simulink model "IOControls"  (R2019b)
settings: configuration reference "ConfigSet_IOControls_Reference" (kept outside this file)
model workspace (MAT data in the model file):
  SampleTime = 0.05
libraries: IOStateMachinesLib x274, SignalGeneratorsLib x1, simulink x1
(part 3 of 10)

== system IOControls/ForEachVehicle/IOControls/Non-CabControl/EDBPanel ==
  ModelInputs : Inport
  Initialise : Inport  Port=2
  BC_Inputs : BusCreator  Inputs=3
  BC_MCBTrip : BusCreator  Inputs=1
  BS_Control1 : BusSelector  OutputSignals=PantographIsolationCock
  BS_Control2 : BusSelector  OutputSignals=VCBIsolationCock
  BS_Control3 : BusSelector  OutputSignals=ORDPlunger
  MCBTripGround : Ground
  ORDPlunger : Subsystem  mask{InitState=0, ControlStates=[0,1], OnStateValue=1, OffStateValue=0}
      mask prompts: InitState "Initial State"; ControlStates "Software State Values"; OnStateValue "On State Value"; OffStateValue "Off State Value"
  PantographIsolationCock : Subsystem  mask{InitState=1, ControlStates=[0,1], OnStateValue=1, OffStateValue=0}
      mask prompts: InitState "Initial State"; ControlStates "Software State Values"; OnStateValue "On State Value"; OffStateValue "Off State Value"
  VCBIsolationCock : Subsystem  mask{InitState=1, ControlStates=[0,1], OnStateValue=1, OffStateValue=0}
      mask prompts: InitState "Initial State"; ControlStates "Software State Values"; OnStateValue "On State Value"; OffStateValue "Off State Value"
  TierControlsInputs : Outport  VectorParamsAs1DForOutWhenUnconnected=off
  TierControlsMCBTrip : Outport  Port=2  VectorParamsAs1DForOutWhenUnconnected=off
  wires:
  MCBTripGround/1 -> BC_MCBTrip/1
  BC_MCBTrip/1 -> TierControlsMCBTrip/1  "EDBPanel"
  BC_Inputs/1 -> TierControlsInputs/1  "EDBPanel"
  ModelInputs/1 -> BS_Control1/1, BS_Control2/1, BS_Control3/1
  BS_Control1/1 -> PantographIsolationCock/1(InputControl)  "<PantographIsolationCock>"
  Initialise/1 -> PantographIsolationCock/2(Initialise), VCBIsolationCock/2(Initialise), ORDPlunger/2(Initialise)
  PantographIsolationCock/1(InputState) -> BC_Inputs/1  "PantographIsolationCock"
  BS_Control2/1 -> VCBIsolationCock/1(InputControl)  "<VCBIsolationCock>"
  VCBIsolationCock/1(InputState) -> BC_Inputs/2  "VCBIsolationCock"
  BS_Control3/1 -> ORDPlunger/1(InputControl)  "<ORDPlunger>"
  ORDPlunger/1(InputState) -> BC_Inputs/3  "ORDPlunger"

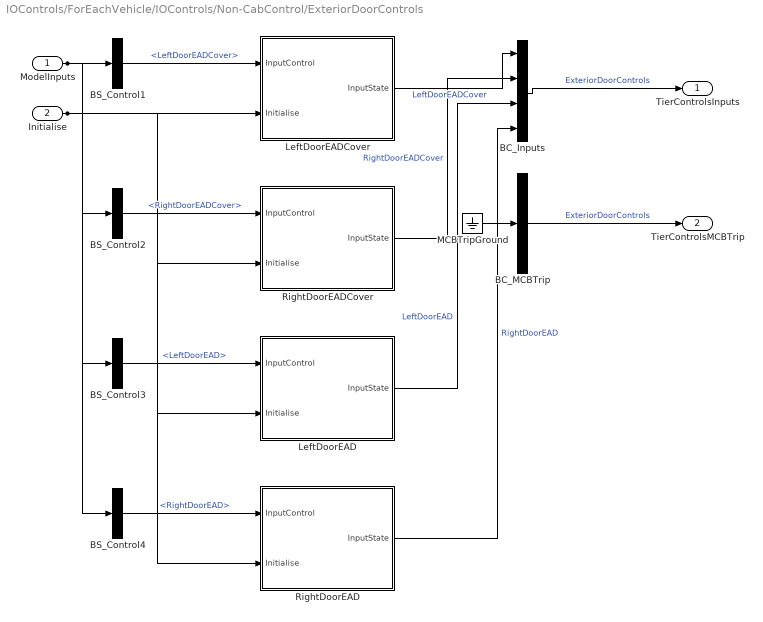
== system IOControls/ForEachVehicle/IOControls/Non-CabControl/ExteriorDoorControls ==
  ModelInputs : Inport
  Initialise : Inport  Port=2
  BC_Inputs : BusCreator  Inputs=4
  BC_MCBTrip : BusCreator  Inputs=1
  BS_Control1 : BusSelector  OutputSignals=LeftDoorEADCover
  BS_Control2 : BusSelector  OutputSignals=RightDoorEADCover
  BS_Control3 : BusSelector  OutputSignals=LeftDoorEAD
  BS_Control4 : BusSelector  OutputSignals=RightDoorEAD
  LeftDoorEAD : Subsystem  mask{InitState=0, ControlStates=[0,1], OnStateValue=1, OffStateValue=0}
      mask prompts: InitState "Initial State"; ControlStates "Software State Values"; OnStateValue "On State Value"; OffStateValue "Off State Value"
  LeftDoorEADCover : Subsystem  mask{InitState=0, ControlStates=[0,1], OnStateValue=1, OffStateValue=0}
      mask prompts: InitState "Initial State"; ControlStates "Software State Values"; OnStateValue "On State Value"; OffStateValue "Off State Value"
  MCBTripGround : Ground
  RightDoorEAD : Subsystem  mask{InitState=0, ControlStates=[0,1], OnStateValue=1, OffStateValue=0}
      mask prompts: InitState "Initial State"; ControlStates "Software State Values"; OnStateValue "On State Value"; OffStateValue "Off State Value"
  RightDoorEADCover : Subsystem  mask{InitState=0, ControlStates=[0,1], OnStateValue=1, OffStateValue=0}
      mask prompts: InitState "Initial State"; ControlStates "Software State Values"; OnStateValue "On State Value"; OffStateValue "Off State Value"
  TierControlsInputs : Outport  VectorParamsAs1DForOutWhenUnconnected=off
  TierControlsMCBTrip : Outport  Port=2  VectorParamsAs1DForOutWhenUnconnected=off
  wires:
  MCBTripGround/1 -> BC_MCBTrip/1
  BC_MCBTrip/1 -> TierControlsMCBTrip/1  "ExteriorDoorControls"
  BC_Inputs/1 -> TierControlsInputs/1  "ExteriorDoorControls"
  ModelInputs/1 -> BS_Control1/1, BS_Control2/1, BS_Control3/1, BS_Control4/1
  BS_Control1/1 -> LeftDoorEADCover/1(InputControl)  "<LeftDoorEADCover>"
  Initialise/1 -> LeftDoorEADCover/2(Initialise), RightDoorEADCover/2(Initialise), LeftDoorEAD/2(Initialise), RightDoorEAD/2(Initialise)
  LeftDoorEADCover/1(InputState) -> BC_Inputs/1  "LeftDoorEADCover"
  BS_Control2/1 -> RightDoorEADCover/1(InputControl)  "<RightDoorEADCover>"
  RightDoorEADCover/1(InputState) -> BC_Inputs/2  "RightDoorEADCover"
  BS_Control3/1 -> LeftDoorEAD/1(InputControl)  "<LeftDoorEAD>"
  LeftDoorEAD/1(InputState) -> BC_Inputs/3  "LeftDoorEAD"
  BS_Control4/1 -> RightDoorEAD/1(InputControl)  "<RightDoorEAD>"
  RightDoorEAD/1(InputState) -> BC_Inputs/4  "RightDoorEAD"

== system IOControls/ForEachVehicle/IOControls/Non-CabControl/ExteriorLights ==
  ModelInputs : Inport
  Initialise : Inport  Port=2
  BC_Inputs : BusCreator  Inputs=1
  BC_MCBTrip : BusCreator  Inputs=1
  InitialiseTerminator : Terminator
  InputsGround : Ground
  MCBTripGround : Ground
  ModelInputsTerminator : Terminator
  TierControlsInputs : Outport  VectorParamsAs1DForOutWhenUnconnected=off
  TierControlsMCBTrip : Outport  Port=2  VectorParamsAs1DForOutWhenUnconnected=off
  wires:
  MCBTripGround/1 -> BC_MCBTrip/1
  InputsGround/1 -> BC_Inputs/1
  Initialise/1 -> InitialiseTerminator/1
  ModelInputs/1 -> ModelInputsTerminator/1
  BC_MCBTrip/1 -> TierControlsMCBTrip/1  "ExteriorLights"
  BC_Inputs/1 -> TierControlsInputs/1  "ExteriorLights"

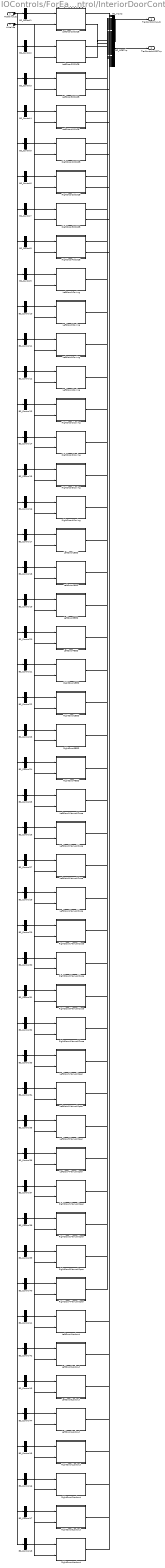
== system IOControls/ForEachVehicle/IOControls/Non-CabControl/InteriorDoorControls ==
  ModelInputs : Inport
  Initialise : Inport  Port=2
  BC_Inputs : BusCreator  Inputs=48
  BC_MCBTrip : BusCreator  Inputs=8
  BS_Control1 : BusSelector  OutputSignals=LeftDoor1DCUCB
  BS_Control10 : BusSelector  OutputSignals=LeftDoor2Coving
  BS_Control11 : BusSelector  OutputSignals=LeftDoor3Coving
  BS_Control12 : BusSelector  OutputSignals=LeftDoor4Coving
  BS_Control13 : BusSelector  OutputSignals=RightDoor1Coving
  BS_Control14 : BusSelector  OutputSignals=RightDoor2Coving
  BS_Control15 : BusSelector  OutputSignals=RightDoor3Coving
  BS_Control16 : BusSelector  OutputSignals=RightDoor4Coving
  BS_Control17 : BusSelector  OutputSignals=LeftDoor1EED
  BS_Control18 : BusSelector  OutputSignals=LeftDoor2EED
  BS_Control19 : BusSelector  OutputSignals=LeftDoor3EED
  BS_Control2 : BusSelector  OutputSignals=LeftDoor2DCUCB
  BS_Control20 : BusSelector  OutputSignals=LeftDoor4EED
  BS_Control21 : BusSelector  OutputSignals=RightDoor1EED
  BS_Control22 : BusSelector  OutputSignals=RightDoor2EED
  BS_Control23 : BusSelector  OutputSignals=RightDoor3EED
  BS_Control24 : BusSelector  OutputSignals=RightDoor4EED
  BS_Control25 : BusSelector  OutputSignals=LeftDoor1ManualClose
  BS_Control26 : BusSelector  OutputSignals=LeftDoor2ManualClose
  BS_Control27 : BusSelector  OutputSignals=LeftDoor3ManualClose
  BS_Control28 : BusSelector  OutputSignals=LeftDoor4ManualClose
  BS_Control29 : BusSelector  OutputSignals=RightDoor1ManualClose
  BS_Control3 : BusSelector  OutputSignals=LeftDoor3DCUCB
  BS_Control30 : BusSelector  OutputSignals=RightDoor2ManualClose
  BS_Control31 : BusSelector  OutputSignals=RightDoor3ManualClose
  BS_Control32 : BusSelector  OutputSignals=RightDoor4ManualClose
  BS_Control33 : BusSelector  OutputSignals=LeftDoor1ManualOpen
  BS_Control34 : BusSelector  OutputSignals=LeftDoor2ManualOpen
  BS_Control35 : BusSelector  OutputSignals=LeftDoor3ManualOpen
  BS_Control36 : BusSelector  OutputSignals=LeftDoor4ManualOpen
  BS_Control37 : BusSelector  OutputSignals=RightDoor1ManualOpen
  BS_Control38 : BusSelector  OutputSignals=RightDoor2ManualOpen
  BS_Control39 : BusSelector  OutputSignals=RightDoor3ManualOpen
  BS_Control4 : BusSelector  OutputSignals=LeftDoor4DCUCB
  BS_Control40 : BusSelector  OutputSignals=RightDoor4ManualOpen
  BS_Control41 : BusSelector  OutputSignals=LeftDoor1Lockout
  BS_Control42 : BusSelector  OutputSignals=LeftDoor2Lockout
  BS_Control43 : BusSelector  OutputSignals=LeftDoor3Lockout
  BS_Control44 : BusSelector  OutputSignals=LeftDoor4Lockout
  BS_Control45 : BusSelector  OutputSignals=RightDoor1Lockout
  BS_Control46 : BusSelector  OutputSignals=RightDoor2Lockout
  BS_Control47 : BusSelector  OutputSignals=RightDoor3Lockout
  BS_Control48 : BusSelector  OutputSignals=RightDoor4Lockout
  BS_Control5 : BusSelector  OutputSignals=RightDoor1DCUCB
  BS_Control6 : BusSelector  OutputSignals=RightDoor2DCUCB
  BS_Control7 : BusSelector  OutputSignals=RightDoor3DCUCB
  BS_Control8 : BusSelector  OutputSignals=RightDoor4DCUCB
  BS_Control9 : BusSelector  OutputSignals=LeftDoor1Coving
  LeftDoor1Coving : Subsystem  mask{InitState=0, ControlStates=[0,1], OnStateValue=1, OffStateValue=0}
      mask prompts: InitState "Initial State"; ControlStates "Software State Values"; OnStateValue "On State Value"; OffStateValue "Off State Value"
  LeftDoor1DCUCB : Subsystem  mask{InitState=1, ControlStates=[0,1], OnStateValue=1, OffStateValue=0}
      mask prompts: InitState "Initial State"; ControlStates "Software State Values"; OnStateValue "On State Value"; OffStateValue "Off State Value"
  LeftDoor1EED : Subsystem  mask{InitState=0, ControlStates=[0,1], OnStateValue=1, OffStateValue=0}
      mask prompts: InitState "Initial State"; ControlStates "Software State Values"; OnStateValue "On State Value"; OffStateValue "Off State Value"
  LeftDoor1Lockout : Subsystem  mask{InitState=0, ControlStates=[0,1], OnStateValue=1, OffStateValue=0}
      mask prompts: InitState "Initial State"; ControlStates "Software State Values"; OnStateValue "On State Value"; OffStateValue "Off State Value"
  LeftDoor1ManualClose : Subsystem  mask{InitState=0, ControlStates=[0,1], OnStateValue=1, OffStateValue=0}
      mask prompts: InitState "Initial State"; ControlStates "Software State Values"; OnStateValue "On State Value"; OffStateValue "Off State Value"
  LeftDoor1ManualOpen : Subsystem  mask{InitState=0, ControlStates=[0,1], OnStateValue=1, OffStateValue=0}
      mask prompts: InitState "Initial State"; ControlStates "Software State Values"; OnStateValue "On State Value"; OffStateValue "Off State Value"
  LeftDoor2Coving : Subsystem  mask{InitState=0, ControlStates=[0,1], OnStateValue=1, OffStateValue=0}
      mask prompts: InitState "Initial State"; ControlStates "Software State Values"; OnStateValue "On State Value"; OffStateValue "Off State Value"
  LeftDoor2DCUCB : Subsystem  mask{InitState=1, ControlStates=[0,1], OnStateValue=1, OffStateValue=0}
      mask prompts: InitState "Initial State"; ControlStates "Software State Values"; OnStateValue "On State Value"; OffStateValue "Off State Value"
  LeftDoor2EED : Subsystem  mask{InitState=0, ControlStates=[0,1], OnStateValue=1, OffStateValue=0}
      mask prompts: InitState "Initial State"; ControlStates "Software State Values"; OnStateValue "On State Value"; OffStateValue "Off State Value"
  LeftDoor2Lockout : Subsystem  mask{InitState=0, ControlStates=[0,1], OnStateValue=1, OffStateValue=0}
      mask prompts: InitState "Initial State"; ControlStates "Software State Values"; OnStateValue "On State Value"; OffStateValue "Off State Value"
  LeftDoor2ManualClose : Subsystem  mask{InitState=0, ControlStates=[0,1], OnStateValue=1, OffStateValue=0}
      mask prompts: InitState "Initial State"; ControlStates "Software State Values"; OnStateValue "On State Value"; OffStateValue "Off State Value"
  LeftDoor2ManualOpen : Subsystem  mask{InitState=0, ControlStates=[0,1], OnStateValue=1, OffStateValue=0}
      mask prompts: InitState "Initial State"; ControlStates "Software State Values"; OnStateValue "On State Value"; OffStateValue "Off State Value"
  LeftDoor3Coving : Subsystem  mask{InitState=0, ControlStates=[0,1], OnStateValue=1, OffStateValue=0}
      mask prompts: InitState "Initial State"; ControlStates "Software State Values"; OnStateValue "On State Value"; OffStateValue "Off State Value"
  LeftDoor3DCUCB : Subsystem  mask{InitState=1, ControlStates=[0,1], OnStateValue=1, OffStateValue=0}
      mask prompts: InitState "Initial State"; ControlStates "Software State Values"; OnStateValue "On State Value"; OffStateValue "Off State Value"
  LeftDoor3EED : Subsystem  mask{InitState=0, ControlStates=[0,1], OnStateValue=1, OffStateValue=0}
      mask prompts: InitState "Initial State"; ControlStates "Software State Values"; OnStateValue "On State Value"; OffStateValue "Off State Value"
  LeftDoor3Lockout : Subsystem  mask{InitState=0, ControlStates=[0,1], OnStateValue=1, OffStateValue=0}
      mask prompts: InitState "Initial State"; ControlStates "Software State Values"; OnStateValue "On State Value"; OffStateValue "Off State Value"
  LeftDoor3ManualClose : Subsystem  mask{InitState=0, ControlStates=[0,1], OnStateValue=1, OffStateValue=0}
      mask prompts: InitState "Initial State"; ControlStates "Software State Values"; OnStateValue "On State Value"; OffStateValue "Off State Value"
  LeftDoor3ManualOpen : Subsystem  mask{InitState=0, ControlStates=[0,1], OnStateValue=1, OffStateValue=0}
      mask prompts: InitState "Initial State"; ControlStates "Software State Values"; OnStateValue "On State Value"; OffStateValue "Off State Value"
  LeftDoor4Coving : Subsystem  mask{InitState=0, ControlStates=[0,1], OnStateValue=1, OffStateValue=0}
      mask prompts: InitState "Initial State"; ControlStates "Software State Values"; OnStateValue "On State Value"; OffStateValue "Off State Value"
  LeftDoor4DCUCB : Subsystem  mask{InitState=1, ControlStates=[0,1], OnStateValue=1, OffStateValue=0}
      mask prompts: InitState "Initial State"; ControlStates "Software State Values"; OnStateValue "On State Value"; OffStateValue "Off State Value"
  LeftDoor4EED : Subsystem  mask{InitState=0, ControlStates=[0,1], OnStateValue=1, OffStateValue=0}
      mask prompts: InitState "Initial State"; ControlStates "Software State Values"; OnStateValue "On State Value"; OffStateValue "Off State Value"
  LeftDoor4Lockout : Subsystem  mask{InitState=0, ControlStates=[0,1], OnStateValue=1, OffStateValue=0}
      mask prompts: InitState "Initial State"; ControlStates "Software State Values"; OnStateValue "On State Value"; OffStateValue "Off State Value"
  LeftDoor4ManualClose : Subsystem  mask{InitState=0, ControlStates=[0,1], OnStateValue=1, OffStateValue=0}
      mask prompts: InitState "Initial State"; ControlStates "Software State Values"; OnStateValue "On State Value"; OffStateValue "Off State Value"
  LeftDoor4ManualOpen : Subsystem  mask{InitState=0, ControlStates=[0,1], OnStateValue=1, OffStateValue=0}
      mask prompts: InitState "Initial State"; ControlStates "Software State Values"; OnStateValue "On State Value"; OffStateValue "Off State Value"
  RightDoor1Coving : Subsystem  mask{InitState=0, ControlStates=[0,1], OnStateValue=1, OffStateValue=0}
      mask prompts: InitState "Initial State"; ControlStates "Software State Values"; OnStateValue "On State Value"; OffStateValue "Off State Value"
  RightDoor1DCUCB : Subsystem  mask{InitState=1, ControlStates=[0,1], OnStateValue=1, OffStateValue=0}
      mask prompts: InitState "Initial State"; ControlStates "Software State Values"; OnStateValue "On State Value"; OffStateValue "Off State Value"
  RightDoor1EED : Subsystem  mask{InitState=0, ControlStates=[0,1], OnStateValue=1, OffStateValue=0}
      mask prompts: InitState "Initial State"; ControlStates "Software State Values"; OnStateValue "On State Value"; OffStateValue "Off State Value"
  RightDoor1Lockout : Subsystem  mask{InitState=0, ControlStates=[0,1], OnStateValue=1, OffStateValue=0}
      mask prompts: InitState "Initial State"; ControlStates "Software State Values"; OnStateValue "On State Value"; OffStateValue "Off State Value"
  RightDoor1ManualClose : Subsystem  mask{InitState=0, ControlStates=[0,1], OnStateValue=1, OffStateValue=0}
      mask prompts: InitState "Initial State"; ControlStates "Software State Values"; OnStateValue "On State Value"; OffStateValue "Off State Value"
  RightDoor1ManualOpen : Subsystem  mask{InitState=0, ControlStates=[0,1], OnStateValue=1, OffStateValue=0}
      mask prompts: InitState "Initial State"; ControlStates "Software State Values"; OnStateValue "On State Value"; OffStateValue "Off State Value"
  RightDoor2Coving : Subsystem  mask{InitState=0, ControlStates=[0,1], OnStateValue=1, OffStateValue=0}
      mask prompts: InitState "Initial State"; ControlStates "Software State Values"; OnStateValue "On State Value"; OffStateValue "Off State Value"
  RightDoor2DCUCB : Subsystem  mask{InitState=1, ControlStates=[0,1], OnStateValue=1, OffStateValue=0}
      mask prompts: InitState "Initial State"; ControlStates "Software State Values"; OnStateValue "On State Value"; OffStateValue "Off State Value"
  RightDoor2EED : Subsystem  mask{InitState=0, ControlStates=[0,1], OnStateValue=1, OffStateValue=0}
      mask prompts: InitState "Initial State"; ControlStates "Software State Values"; OnStateValue "On State Value"; OffStateValue "Off State Value"
  RightDoor2Lockout : Subsystem  mask{InitState=0, ControlStates=[0,1], OnStateValue=1, OffStateValue=0}
      mask prompts: InitState "Initial State"; ControlStates "Software State Values"; OnStateValue "On State Value"; OffStateValue "Off State Value"
  RightDoor2ManualClose : Subsystem  mask{InitState=0, ControlStates=[0,1], OnStateValue=1, OffStateValue=0}
      mask prompts: InitState "Initial State"; ControlStates "Software State Values"; OnStateValue "On State Value"; OffStateValue "Off State Value"
  RightDoor2ManualOpen : Subsystem  mask{InitState=0, ControlStates=[0,1], OnStateValue=1, OffStateValue=0}
      mask prompts: InitState "Initial State"; ControlStates "Software State Values"; OnStateValue "On State Value"; OffStateValue "Off State Value"
  RightDoor3Coving : Subsystem  mask{InitState=0, ControlStates=[0,1], OnStateValue=1, OffStateValue=0}
      mask prompts: InitState "Initial State"; ControlStates "Software State Values"; OnStateValue "On State Value"; OffStateValue "Off State Value"
  RightDoor3DCUCB : Subsystem  mask{InitState=1, ControlStates=[0,1], OnStateValue=1, OffStateValue=0}
      mask prompts: InitState "Initial State"; ControlStates "Software State Values"; OnStateValue "On State Value"; OffStateValue "Off State Value"
  RightDoor3EED : Subsystem  mask{InitState=0, ControlStates=[0,1], OnStateValue=1, OffStateValue=0}
      mask prompts: InitState "Initial State"; ControlStates "Software State Values"; OnStateValue "On State Value"; OffStateValue "Off State Value"
  RightDoor3Lockout : Subsystem  mask{InitState=0, ControlStates=[0,1], OnStateValue=1, OffStateValue=0}
      mask prompts: InitState "Initial State"; ControlStates "Software State Values"; OnStateValue "On State Value"; OffStateValue "Off State Value"
  RightDoor3ManualClose : Subsystem  mask{InitState=0, ControlStates=[0,1], OnStateValue=1, OffStateValue=0}
      mask prompts: InitState "Initial State"; ControlStates "Software State Values"; OnStateValue "On State Value"; OffStateValue "Off State Value"
  RightDoor3ManualOpen : Subsystem  mask{InitState=0, ControlStates=[0,1], OnStateValue=1, OffStateValue=0}
      mask prompts: InitState "Initial State"; ControlStates "Software State Values"; OnStateValue "On State Value"; OffStateValue "Off State Value"
  RightDoor4Coving : Subsystem  mask{InitState=0, ControlStates=[0,1], OnStateValue=1, OffStateValue=0}
      mask prompts: InitState "Initial State"; ControlStates "Software State Values"; OnStateValue "On State Value"; OffStateValue "Off State Value"
  RightDoor4DCUCB : Subsystem  mask{InitState=1, ControlStates=[0,1], OnStateValue=1, OffStateValue=0}
      mask prompts: InitState "Initial State"; ControlStates "Software State Values"; OnStateValue "On State Value"; OffStateValue "Off State Value"
  RightDoor4EED : Subsystem  mask{InitState=0, ControlStates=[0,1], OnStateValue=1, OffStateValue=0}
      mask prompts: InitState "Initial State"; ControlStates "Software State Values"; OnStateValue "On State Value"; OffStateValue "Off State Value"
  RightDoor4Lockout : Subsystem  mask{InitState=0, ControlStates=[0,1], OnStateValue=1, OffStateValue=0}
      mask prompts: InitState "Initial State"; ControlStates "Software State Values"; OnStateValue "On State Value"; OffStateValue "Off State Value"
  RightDoor4ManualClose : Subsystem  mask{InitState=0, ControlStates=[0,1], OnStateValue=1, OffStateValue=0}
      mask prompts: InitState "Initial State"; ControlStates "Software State Values"; OnStateValue "On State Value"; OffStateValue "Off State Value"
  RightDoor4ManualOpen : Subsystem  mask{InitState=0, ControlStates=[0,1], OnStateValue=1, OffStateValue=0}
      mask prompts: InitState "Initial State"; ControlStates "Software State Values"; OnStateValue "On State Value"; OffStateValue "Off State Value"
  TierControlsInputs : Outport  VectorParamsAs1DForOutWhenUnconnected=off
  TierControlsMCBTrip : Outport  Port=2  VectorParamsAs1DForOutWhenUnconnected=off
  wires:
  BC_MCBTrip/1 -> TierControlsMCBTrip/1  "InteriorDoorControls"
  BC_Inputs/1 -> TierControlsInputs/1  "InteriorDoorControls"
  ModelInputs/1 -> BS_Control1/1, BS_Control2/1, BS_Control3/1, BS_Control4/1, BS_Control5/1, BS_Control6/1, BS_Control7/1, BS_Control8/1, BS_Control9/1, BS_Control10/1, BS_Control11/1, BS_Control12/1, BS_Control13/1, BS_Control14/1, BS_Control15/1, BS_Control16/1, BS_Control17/1, BS_Control18/1, BS_Control19/1, BS_Control20/1, BS_Control21/1, BS_Control22/1, BS_Control23/1, BS_Control24/1, BS_Control25/1, BS_Control26/1, BS_Control27/1, BS_Control28/1, BS_Control29/1, BS_Control30/1, BS_Control31/1, BS_Control32/1, BS_Control33/1, BS_Control34/1, BS_Control35/1, BS_Control36/1, BS_Control37/1, BS_Control38/1, BS_Control39/1, BS_Control40/1, BS_Control41/1, BS_Control42/1, BS_Control43/1, BS_Control44/1, BS_Control45/1, BS_Control46/1, BS_Control47/1, BS_Control48/1
  BS_Control1/1 -> LeftDoor1DCUCB/1(MCBControl)  "<LeftDoor1DCUCB>"
  Initialise/1 -> LeftDoor1DCUCB/2(Initialise), LeftDoor2DCUCB/2(Initialise), LeftDoor3DCUCB/2(Initialise), LeftDoor4DCUCB/2(Initialise), RightDoor1DCUCB/2(Initialise), RightDoor2DCUCB/2(Initialise), RightDoor3DCUCB/2(Initialise), RightDoor4DCUCB/2(Initialise), LeftDoor1Coving/2(Initialise), LeftDoor2Coving/2(Initialise), LeftDoor3Coving/2(Initialise), LeftDoor4Coving/2(Initialise), RightDoor1Coving/2(Initialise), RightDoor2Coving/2(Initialise), RightDoor3Coving/2(Initialise), RightDoor4Coving/2(Initialise), LeftDoor1EED/2(Initialise), LeftDoor2EED/2(Initialise), LeftDoor3EED/2(Initialise), LeftDoor4EED/2(Initialise), RightDoor1EED/2(Initialise), RightDoor2EED/2(Initialise), RightDoor3EED/2(Initialise), RightDoor4EED/2(Initialise), LeftDoor1ManualClose/2(Initialise), LeftDoor2ManualClose/2(Initialise), LeftDoor3ManualClose/2(Initialise), LeftDoor4ManualClose/2(Initialise), RightDoor1ManualClose/2(Initialise), RightDoor2ManualClose/2(Initialise), RightDoor3ManualClose/2(Initialise), RightDoor4ManualClose/2(Initialise), LeftDoor1ManualOpen/2(Initialise), LeftDoor2ManualOpen/2(Initialise), LeftDoor3ManualOpen/2(Initialise), LeftDoor4ManualOpen/2(Initialise), RightDoor1ManualOpen/2(Initialise), RightDoor2ManualOpen/2(Initialise), RightDoor3ManualOpen/2(Initialise), RightDoor4ManualOpen/2(Initialise), LeftDoor1Lockout/2(Initialise), LeftDoor2Lockout/2(Initialise), LeftDoor3Lockout/2(Initialise), LeftDoor4Lockout/2(Initialise), RightDoor1Lockout/2(Initialise), RightDoor2Lockout/2(Initialise), RightDoor3Lockout/2(Initialise), RightDoor4Lockout/2(Initialise)
  LeftDoor1DCUCB/1(InputState) -> BC_Inputs/1  "LeftDoor1DCUCB"
  LeftDoor1DCUCB/2(MCBTripState) -> BC_MCBTrip/1  "LeftDoor1DCUCB"
  BS_Control2/1 -> LeftDoor2DCUCB/1(MCBControl)  "<LeftDoor2DCUCB>"
  LeftDoor2DCUCB/1(InputState) -> BC_Inputs/2  "LeftDoor2DCUCB"
  LeftDoor2DCUCB/2(MCBTripState) -> BC_MCBTrip/2  "LeftDoor2DCUCB"
  BS_Control3/1 -> LeftDoor3DCUCB/1(MCBControl)  "<LeftDoor3DCUCB>"
  LeftDoor3DCUCB/1(InputState) -> BC_Inputs/3  "LeftDoor3DCUCB"
  LeftDoor3DCUCB/2(MCBTripState) -> BC_MCBTrip/3  "LeftDoor3DCUCB"
  BS_Control4/1 -> LeftDoor4DCUCB/1(MCBControl)  "<LeftDoor4DCUCB>"
  LeftDoor4DCUCB/1(InputState) -> BC_Inputs/4  "LeftDoor4DCUCB"
  LeftDoor4DCUCB/2(MCBTripState) -> BC_MCBTrip/4  "LeftDoor4DCUCB"
  BS_Control5/1 -> RightDoor1DCUCB/1(MCBControl)  "<RightDoor1DCUCB>"
  RightDoor1DCUCB/1(InputState) -> BC_Inputs/5  "RightDoor1DCUCB"
  RightDoor1DCUCB/2(MCBTripState) -> BC_MCBTrip/5  "RightDoor1DCUCB"
  BS_Control6/1 -> RightDoor2DCUCB/1(MCBControl)  "<RightDoor2DCUCB>"
  RightDoor2DCUCB/1(InputState) -> BC_Inputs/6  "RightDoor2DCUCB"
  RightDoor2DCUCB/2(MCBTripState) -> BC_MCBTrip/6  "RightDoor2DCUCB"
  BS_Control7/1 -> RightDoor3DCUCB/1(MCBControl)  "<RightDoor3DCUCB>"
  RightDoor3DCUCB/1(InputState) -> BC_Inputs/7  "RightDoor3DCUCB"
  RightDoor3DCUCB/2(MCBTripState) -> BC_MCBTrip/7  "RightDoor3DCUCB"
  BS_Control8/1 -> RightDoor4DCUCB/1(MCBControl)  "<RightDoor4DCUCB>"
  RightDoor4DCUCB/1(InputState) -> BC_Inputs/8  "RightDoor4DCUCB"
  RightDoor4DCUCB/2(MCBTripState) -> BC_MCBTrip/8  "RightDoor4DCUCB"
  BS_Control9/1 -> LeftDoor1Coving/1(InputControl)  "<LeftDoor1Coving>"
  LeftDoor1Coving/1(InputState) -> BC_Inputs/9  "LeftDoor1Coving"
  BS_Control10/1 -> LeftDoor2Coving/1(InputControl)  "<LeftDoor2Coving>"
  LeftDoor2Coving/1(InputState) -> BC_Inputs/10  "LeftDoor2Coving"
  BS_Control11/1 -> LeftDoor3Coving/1(InputControl)  "<LeftDoor3Coving>"
  LeftDoor3Coving/1(InputState) -> BC_Inputs/11  "LeftDoor3Coving"
  BS_Control12/1 -> LeftDoor4Coving/1(InputControl)  "<LeftDoor4Coving>"
  LeftDoor4Coving/1(InputState) -> BC_Inputs/12  "LeftDoor4Coving"
  BS_Control13/1 -> RightDoor1Coving/1(InputControl)  "<RightDoor1Coving>"
  RightDoor1Coving/1(InputState) -> BC_Inputs/13  "RightDoor1Coving"
  BS_Control14/1 -> RightDoor2Coving/1(InputControl)  "<RightDoor2Coving>"
  RightDoor2Coving/1(InputState) -> BC_Inputs/14  "RightDoor2Coving"
  BS_Control15/1 -> RightDoor3Coving/1(InputControl)  "<RightDoor3Coving>"
  RightDoor3Coving/1(InputState) -> BC_Inputs/15  "RightDoor3Coving"
  BS_Control16/1 -> RightDoor4Coving/1(InputControl)  "<RightDoor4Coving>"
  RightDoor4Coving/1(InputState) -> BC_Inputs/16  "RightDoor4Coving"
  BS_Control17/1 -> LeftDoor1EED/1(InputControl)  "<LeftDoor1EED>"
  LeftDoor1EED/1(InputState) -> BC_Inputs/17  "LeftDoor1EED"
  BS_Control18/1 -> LeftDoor2EED/1(InputControl)  "<LeftDoor2EED>"
  LeftDoor2EED/1(InputState) -> BC_Inputs/18  "LeftDoor2EED"
  BS_Control19/1 -> LeftDoor3EED/1(InputControl)  "<LeftDoor3EED>"
  LeftDoor3EED/1(InputState) -> BC_Inputs/19  "LeftDoor3EED"
  BS_Control20/1 -> LeftDoor4EED/1(InputControl)  "<LeftDoor4EED>"
  LeftDoor4EED/1(InputState) -> BC_Inputs/20  "LeftDoor4EED"
  BS_Control21/1 -> RightDoor1EED/1(InputControl)  "<RightDoor1EED>"
  RightDoor1EED/1(InputState) -> BC_Inputs/21  "RightDoor1EED"
  BS_Control22/1 -> RightDoor2EED/1(InputControl)  "<RightDoor2EED>"
  RightDoor2EED/1(InputState) -> BC_Inputs/22  "RightDoor2EED"
  BS_Control23/1 -> RightDoor3EED/1(InputControl)  "<RightDoor3EED>"
  RightDoor3EED/1(InputState) -> BC_Inputs/23  "RightDoor3EED"
  BS_Control24/1 -> RightDoor4EED/1(InputControl)  "<RightDoor4EED>"
  RightDoor4EED/1(InputState) -> BC_Inputs/24  "RightDoor4EED"
  BS_Control25/1 -> LeftDoor1ManualClose/1(InputControl)  "<LeftDoor1ManualClose>"
  LeftDoor1ManualClose/1(InputState) -> BC_Inputs/25  "LeftDoor1ManualClose"
  BS_Control26/1 -> LeftDoor2ManualClose/1(InputControl)  "<LeftDoor2ManualClose>"
  LeftDoor2ManualClose/1(InputState) -> BC_Inputs/26  "LeftDoor2ManualClose"
  BS_Control27/1 -> LeftDoor3ManualClose/1(InputControl)  "<LeftDoor3ManualClose>"
  LeftDoor3ManualClose/1(InputState) -> BC_Inputs/27  "LeftDoor3ManualClose"
  BS_Control28/1 -> LeftDoor4ManualClose/1(InputControl)  "<LeftDoor4ManualClose>"
  LeftDoor4ManualClose/1(InputState) -> BC_Inputs/28  "LeftDoor4ManualClose"
  BS_Control29/1 -> RightDoor1ManualClose/1(InputControl)  "<RightDoor1ManualClose>"
  RightDoor1ManualClose/1(InputState) -> BC_Inputs/29  "RightDoor1ManualClose"
  BS_Control30/1 -> RightDoor2ManualClose/1(InputControl)  "<RightDoor2ManualClose>"
  RightDoor2ManualClose/1(InputState) -> BC_Inputs/30  "RightDoor2ManualClose"
  BS_Control31/1 -> RightDoor3ManualClose/1(InputControl)  "<RightDoor3ManualClose>"
  RightDoor3ManualClose/1(InputState) -> BC_Inputs/31  "RightDoor3ManualClose"
  BS_Control32/1 -> RightDoor4ManualClose/1(InputControl)  "<RightDoor4ManualClose>"
  RightDoor4ManualClose/1(InputState) -> BC_Inputs/32  "RightDoor4ManualClose"
  BS_Control33/1 -> LeftDoor1ManualOpen/1(InputControl)  "<LeftDoor1ManualOpen>"
  LeftDoor1ManualOpen/1(InputState) -> BC_Inputs/33  "LeftDoor1ManualOpen"
  BS_Control34/1 -> LeftDoor2ManualOpen/1(InputControl)  "<LeftDoor2ManualOpen>"
  LeftDoor2ManualOpen/1(InputState) -> BC_Inputs/34  "LeftDoor2ManualOpen"
  BS_Control35/1 -> LeftDoor3ManualOpen/1(InputControl)  "<LeftDoor3ManualOpen>"
  LeftDoor3ManualOpen/1(InputState) -> BC_Inputs/35  "LeftDoor3ManualOpen"
  BS_Control36/1 -> LeftDoor4ManualOpen/1(InputControl)  "<LeftDoor4ManualOpen>"
  LeftDoor4ManualOpen/1(InputState) -> BC_Inputs/36  "LeftDoor4ManualOpen"
  BS_Control37/1 -> RightDoor1ManualOpen/1(InputControl)  "<RightDoor1ManualOpen>"
  RightDoor1ManualOpen/1(InputState) -> BC_Inputs/37  "RightDoor1ManualOpen"
  BS_Control38/1 -> RightDoor2ManualOpen/1(InputControl)  "<RightDoor2ManualOpen>"
  RightDoor2ManualOpen/1(InputState) -> BC_Inputs/38  "RightDoor2ManualOpen"
  BS_Control39/1 -> RightDoor3ManualOpen/1(InputControl)  "<RightDoor3ManualOpen>"
  RightDoor3ManualOpen/1(InputState) -> BC_Inputs/39  "RightDoor3ManualOpen"
  BS_Control40/1 -> RightDoor4ManualOpen/1(InputControl)  "<RightDoor4ManualOpen>"
  RightDoor4ManualOpen/1(InputState) -> BC_Inputs/40  "RightDoor4ManualOpen"
  BS_Control41/1 -> LeftDoor1Lockout/1(InputControl)  "<LeftDoor1Lockout>"
  LeftDoor1Lockout/1(InputState) -> BC_Inputs/41  "LeftDoor1Lockout"
  BS_Control42/1 -> LeftDoor2Lockout/1(InputControl)  "<LeftDoor2Lockout>"
  LeftDoor2Lockout/1(InputState) -> BC_Inputs/42  "LeftDoor2Lockout"
  BS_Control43/1 -> LeftDoor3Lockout/1(InputControl)  "<LeftDoor3Lockout>"
  LeftDoor3Lockout/1(InputState) -> BC_Inputs/43  "LeftDoor3Lockout"
  BS_Control44/1 -> LeftDoor4Lockout/1(InputControl)  "<LeftDoor4Lockout>"
  LeftDoor4Lockout/1(InputState) -> BC_Inputs/44  "LeftDoor4Lockout"
  BS_Control45/1 -> RightDoor1Lockout/1(InputControl)  "<RightDoor1Lockout>"
  RightDoor1Lockout/1(InputState) -> BC_Inputs/45  "RightDoor1Lockout"
  BS_Control46/1 -> RightDoor2Lockout/1(InputControl)  "<RightDoor2Lockout>"
  RightDoor2Lockout/1(InputState) -> BC_Inputs/46  "RightDoor2Lockout"
  BS_Control47/1 -> RightDoor3Lockout/1(InputControl)  "<RightDoor3Lockout>"
  RightDoor3Lockout/1(InputState) -> BC_Inputs/47  "RightDoor3Lockout"
  BS_Control48/1 -> RightDoor4Lockout/1(InputControl)  "<RightDoor4Lockout>"
  RightDoor4Lockout/1(InputState) -> BC_Inputs/48  "RightDoor4Lockout"

== system IOControls/ForEachVehicle/IOControls/Non-CabControl/PassengerEmergencyControlUnit ==
  ModelInputs : Inport
  Initialise : Inport  Port=2
  BC_Inputs : BusCreator  Inputs=3
  BC_MCBTrip : BusCreator  Inputs=1
  BS_Control1 : BusSelector  OutputSignals=PECUPushButton
  BS_Control2 : BusSelector  OutputSignals=Microphone
  BS_Control3 : BusSelector  OutputSignals=DriversBackDoor
  DriversBackDoor : Subsystem  mask{InitState=0, ControlStates=[0,1], OnStateValue=1, OffStateValue=0}
      mask prompts: InitState "Initial State"; ControlStates "Software State Values"; OnStateValue "On State Value"; OffStateValue "Off State Value"
  MCBTripGround : Ground
  Microphone : Subsystem  mask{InitState=0, ControlStates=[0,1], OnStateValue=1, OffStateValue=0}
      mask prompts: InitState "Initial State"; ControlStates "Software State Values"; OnStateValue "On State Value"; OffStateValue "Off State Value"
  PECUPushButton : Subsystem  mask{InitState=0, ControlStates=[0,1], OnStateValue=1, OffStateValue=0}
      mask prompts: InitState "Initial State"; ControlStates "Software State Values"; OnStateValue "On State Value"; OffStateValue "Off State Value"
  TierControlsInputs : Outport  VectorParamsAs1DForOutWhenUnconnected=off
  TierControlsMCBTrip : Outport  Port=2  VectorParamsAs1DForOutWhenUnconnected=off
  wires:
  MCBTripGround/1 -> BC_MCBTrip/1
  BC_MCBTrip/1 -> TierControlsMCBTrip/1  "PassengerEmergencyControlUnit"
  BC_Inputs/1 -> TierControlsInputs/1  "PassengerEmergencyControlUnit"
  ModelInputs/1 -> BS_Control1/1, BS_Control2/1, BS_Control3/1
  BS_Control1/1 -> PECUPushButton/1(InputControl)  "<PECUPushButton>"
  Initialise/1 -> PECUPushButton/2(Initialise), Microphone/2(Initialise), DriversBackDoor/2(Initialise)
  PECUPushButton/1(InputState) -> BC_Inputs/1  "PECUPushButton"
  BS_Control2/1 -> Microphone/1(InputControl)  "<Microphone>"
  Microphone/1(InputState) -> BC_Inputs/2  "Microphone"
  BS_Control3/1 -> DriversBackDoor/1(InputControl)  "<DriversBackDoor>"
  DriversBackDoor/1(InputState) -> BC_Inputs/3  "DriversBackDoor"

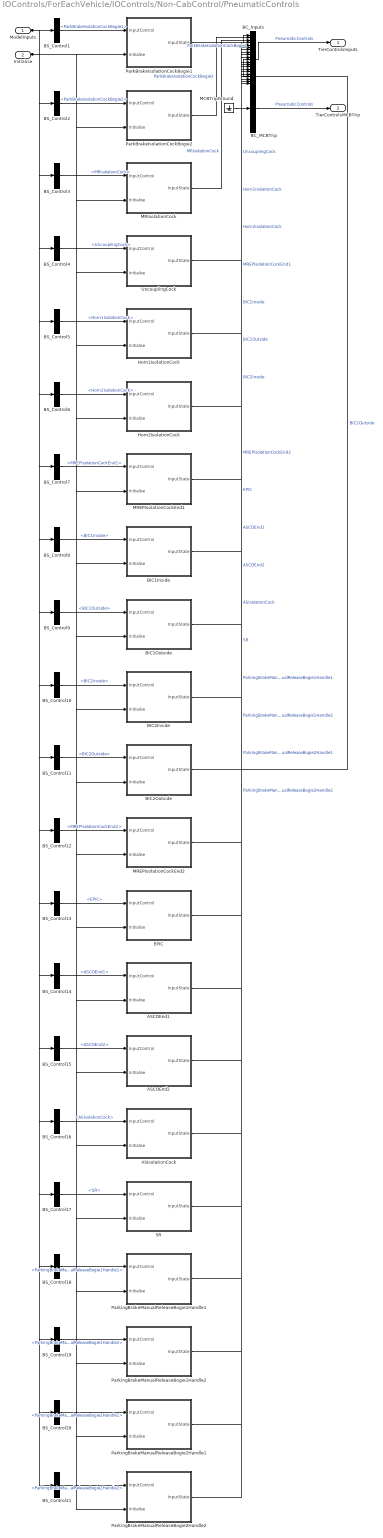
== system IOControls/ForEachVehicle/IOControls/Non-CabControl/PneumaticControls ==
  ModelInputs : Inport
  Initialise : Inport  Port=2
  ASCOEnd1 : Subsystem  mask{InitState=1, ControlStates=[0,1], OnStateValue=1, OffStateValue=0}
      mask prompts: InitState "Initial State"; ControlStates "Software State Values"; OnStateValue "On State Value"; OffStateValue "Off State Value"
  ASCOEnd2 : Subsystem  mask{InitState=1, ControlStates=[0,1], OnStateValue=1, OffStateValue=0}
      mask prompts: InitState "Initial State"; ControlStates "Software State Values"; OnStateValue "On State Value"; OffStateValue "Off State Value"
  ASIsolationCock : Subsystem  mask{InitState=1, ControlStates=[0,1], OnStateValue=1, OffStateValue=0}
      mask prompts: InitState "Initial State"; ControlStates "Software State Values"; OnStateValue "On State Value"; OffStateValue "Off State Value"
  BC_Inputs : BusCreator  Inputs=21
  BC_MCBTrip : BusCreator  Inputs=1
  BIC1Inside : Subsystem  mask{InitState=1, ControlStates=[0,1], OnStateValue=1, OffStateValue=0}
      mask prompts: InitState "Initial State"; ControlStates "Software State Values"; OnStateValue "On State Value"; OffStateValue "Off State Value"
  BIC1Outside : Subsystem  mask{InitState=1, ControlStates=[0,1], OnStateValue=1, OffStateValue=0}
      mask prompts: InitState "Initial State"; ControlStates "Software State Values"; OnStateValue "On State Value"; OffStateValue "Off State Value"
  BIC2Inside : Subsystem  mask{InitState=1, ControlStates=[0,1], OnStateValue=1, OffStateValue=0}
      mask prompts: InitState "Initial State"; ControlStates "Software State Values"; OnStateValue "On State Value"; OffStateValue "Off State Value"
  BIC2Outside : Subsystem  mask{InitState=1, ControlStates=[0,1], OnStateValue=1, OffStateValue=0}
      mask prompts: InitState "Initial State"; ControlStates "Software State Values"; OnStateValue "On State Value"; OffStateValue "Off State Value"
  BS_Control1 : BusSelector  OutputSignals=ParkBrakeIsolationCockBogie1
  BS_Control10 : BusSelector  OutputSignals=BIC2Inside
  BS_Control11 : BusSelector  OutputSignals=BIC2Outside
  BS_Control12 : BusSelector  OutputSignals=MREPIsolationCockEnd2
  BS_Control13 : BusSelector  OutputSignals=EPIC
  BS_Control14 : BusSelector  OutputSignals=ASCOEnd1
  BS_Control15 : BusSelector  OutputSignals=ASCOEnd2
  BS_Control16 : BusSelector  OutputSignals=ASIsolationCock
  BS_Control17 : BusSelector  OutputSignals=SR
  BS_Control18 : BusSelector  OutputSignals=ParkingBrakeManualReleaseBogie1Handle1
  BS_Control19 : BusSelector  OutputSignals=ParkingBrakeManualReleaseBogie1Handle2
  BS_Control2 : BusSelector  OutputSignals=ParkBrakeIsolationCockBogie2
  BS_Control20 : BusSelector  OutputSignals=ParkingBrakeManualReleaseBogie2Handle1
  BS_Control21 : BusSelector  OutputSignals=ParkingBrakeManualReleaseBogie2Handle2
  BS_Control3 : BusSelector  OutputSignals=MRIsolationCock
  BS_Control4 : BusSelector  OutputSignals=UncouplingCock
  BS_Control5 : BusSelector  OutputSignals=Horn1IsolationCock
  BS_Control6 : BusSelector  OutputSignals=Horn2IsolationCock
  BS_Control7 : BusSelector  OutputSignals=MREPIsolationCockEnd1
  BS_Control8 : BusSelector  OutputSignals=BIC1Inside
  BS_Control9 : BusSelector  OutputSignals=BIC1Outside
  EPIC : Subsystem  mask{InitState=1, ControlStates=[0,1], OnStateValue=1, OffStateValue=0}
      mask prompts: InitState "Initial State"; ControlStates "Software State Values"; OnStateValue "On State Value"; OffStateValue "Off State Value"
  Horn1IsolationCock : Subsystem  mask{InitState=1, ControlStates=[0,1], OnStateValue=1, OffStateValue=0}
      mask prompts: InitState "Initial State"; ControlStates "Software State Values"; OnStateValue "On State Value"; OffStateValue "Off State Value"
  Horn2IsolationCock : Subsystem  mask{InitState=1, ControlStates=[0,1], OnStateValue=1, OffStateValue=0}
      mask prompts: InitState "Initial State"; ControlStates "Software State Values"; OnStateValue "On State Value"; OffStateValue "Off State Value"
  MCBTripGround : Ground
  MREPIsolationCockEnd1 : Subsystem  mask{InitState=1, ControlStates=[0,1], OnStateValue=1, OffStateValue=0}
      mask prompts: InitState "Initial State"; ControlStates "Software State Values"; OnStateValue "On State Value"; OffStateValue "Off State Value"
  MREPIsolationCockEnd2 : Subsystem  mask{InitState=1, ControlStates=[0,1], OnStateValue=1, OffStateValue=0}
      mask prompts: InitState "Initial State"; ControlStates "Software State Values"; OnStateValue "On State Value"; OffStateValue "Off State Value"
  MRIsolationCock : Subsystem  mask{InitState=1, ControlStates=[0,1], OnStateValue=1, OffStateValue=0}
      mask prompts: InitState "Initial State"; ControlStates "Software State Values"; OnStateValue "On State Value"; OffStateValue "Off State Value"
  ParkBrakeIsolationCockBogie1 : Subsystem  mask{InitState=1, ControlStates=[0,1], OnStateValue=1, OffStateValue=0}
      mask prompts: InitState "Initial State"; ControlStates "Software State Values"; OnStateValue "On State Value"; OffStateValue "Off State Value"
  ParkBrakeIsolationCockBogie2 : Subsystem  mask{InitState=1, ControlStates=[0,1], OnStateValue=1, OffStateValue=0}
      mask prompts: InitState "Initial State"; ControlStates "Software State Values"; OnStateValue "On State Value"; OffStateValue "Off State Value"
  ParkingBrakeManualReleaseBogie1Handle1 : Subsystem  mask{InitState=0, ControlStates=[0,1], OnStateValue=1, OffStateValue=0}
      mask prompts: InitState "Initial State"; ControlStates "Software State Values"; OnStateValue "On State Value"; OffStateValue "Off State Value"
  ParkingBrakeManualReleaseBogie1Handle2 : Subsystem  mask{InitState=0, ControlStates=[0,1], OnStateValue=1, OffStateValue=0}
      mask prompts: InitState "Initial State"; ControlStates "Software State Values"; OnStateValue "On State Value"; OffStateValue "Off State Value"
  ParkingBrakeManualReleaseBogie2Handle1 : Subsystem  mask{InitState=0, ControlStates=[0,1], OnStateValue=1, OffStateValue=0}
      mask prompts: InitState "Initial State"; ControlStates "Software State Values"; OnStateValue "On State Value"; OffStateValue "Off State Value"
  ParkingBrakeManualReleaseBogie2Handle2 : Subsystem  mask{InitState=0, ControlStates=[0,1], OnStateValue=1, OffStateValue=0}
      mask prompts: InitState "Initial State"; ControlStates "Software State Values"; OnStateValue "On State Value"; OffStateValue "Off State Value"
  SR : Subsystem  mask{InitState=1, ControlStates=[0,1], OnStateValue=1, OffStateValue=0}
      mask prompts: InitState "Initial State"; ControlStates "Software State Values"; OnStateValue "On State Value"; OffStateValue "Off State Value"
  UncouplingCock : Subsystem  mask{InitState=1, ControlStates=[0,1], OnStateValue=1, OffStateValue=0}
      mask prompts: InitState "Initial State"; ControlStates "Software State Values"; OnStateValue "On State Value"; OffStateValue "Off State Value"
  TierControlsInputs : Outport  VectorParamsAs1DForOutWhenUnconnected=off
  TierControlsMCBTrip : Outport  Port=2  VectorParamsAs1DForOutWhenUnconnected=off
  wires:
  MCBTripGround/1 -> BC_MCBTrip/1
  BC_MCBTrip/1 -> TierControlsMCBTrip/1  "PneumaticControls"
  BC_Inputs/1 -> TierControlsInputs/1  "PneumaticControls"
  ModelInputs/1 -> BS_Control1/1, BS_Control2/1, BS_Control3/1, BS_Control4/1, BS_Control5/1, BS_Control6/1, BS_Control7/1, BS_Control8/1, BS_Control9/1, BS_Control10/1, BS_Control11/1, BS_Control12/1, BS_Control13/1, BS_Control14/1, BS_Control15/1, BS_Control16/1, BS_Control17/1, BS_Control18/1, BS_Control19/1, BS_Control20/1, BS_Control21/1
  BS_Control1/1 -> ParkBrakeIsolationCockBogie1/1(InputControl)  "<ParkBrakeIsolationCockBogie1>"
  Initialise/1 -> ParkBrakeIsolationCockBogie1/2(Initialise), ParkBrakeIsolationCockBogie2/2(Initialise), MRIsolationCock/2(Initialise), UncouplingCock/2(Initialise), Horn1IsolationCock/2(Initialise), Horn2IsolationCock/2(Initialise), MREPIsolationCockEnd1/2(Initialise), BIC1Inside/2(Initialise), BIC1Outside/2(Initialise), BIC2Inside/2(Initialise), BIC2Outside/2(Initialise), MREPIsolationCockEnd2/2(Initialise), EPIC/2(Initialise), ASCOEnd1/2(Initialise), ASCOEnd2/2(Initialise), ASIsolationCock/2(Initialise), SR/2(Initialise), ParkingBrakeManualReleaseBogie1Handle1/2(Initialise), ParkingBrakeManualReleaseBogie1Handle2/2(Initialise), ParkingBrakeManualReleaseBogie2Handle1/2(Initialise), ParkingBrakeManualReleaseBogie2Handle2/2(Initialise)
  ParkBrakeIsolationCockBogie1/1(InputState) -> BC_Inputs/1  "ParkBrakeIsolationCockBogie1"
  BS_Control2/1 -> ParkBrakeIsolationCockBogie2/1(InputControl)  "<ParkBrakeIsolationCockBogie2>"
  ParkBrakeIsolationCockBogie2/1(InputState) -> BC_Inputs/2  "ParkBrakeIsolationCockBogie2"
  BS_Control3/1 -> MRIsolationCock/1(InputControl)  "<MRIsolationCock>"
  MRIsolationCock/1(InputState) -> BC_Inputs/3  "MRIsolationCock"
  BS_Control4/1 -> UncouplingCock/1(InputControl)  "<UncouplingCock>"
  UncouplingCock/1(InputState) -> BC_Inputs/4  "UncouplingCock"
  BS_Control5/1 -> Horn1IsolationCock/1(InputControl)  "<Horn1IsolationCock>"
  Horn1IsolationCock/1(InputState) -> BC_Inputs/5  "Horn1IsolationCock"
  BS_Control6/1 -> Horn2IsolationCock/1(InputControl)  "<Horn2IsolationCock>"
  Horn2IsolationCock/1(InputState) -> BC_Inputs/6  "Horn2IsolationCock"
  BS_Control7/1 -> MREPIsolationCockEnd1/1(InputControl)  "<MREPIsolationCockEnd1>"
  MREPIsolationCockEnd1/1(InputState) -> BC_Inputs/7  "MREPIsolationCockEnd1"
  BS_Control8/1 -> BIC1Inside/1(InputControl)  "<BIC1Inside>"
  BIC1Inside/1(InputState) -> BC_Inputs/8  "BIC1Inside"
  BS_Control9/1 -> BIC1Outside/1(InputControl)  "<BIC1Outside>"
  BIC1Outside/1(InputState) -> BC_Inputs/9  "BIC1Outside"
  BS_Control10/1 -> BIC2Inside/1(InputControl)  "<BIC2Inside>"
  BIC2Inside/1(InputState) -> BC_Inputs/10  "BIC2Inside"
  BS_Control11/1 -> BIC2Outside/1(InputControl)  "<BIC2Outside>"
  BIC2Outside/1(InputState) -> BC_Inputs/11  "BIC2Outside"
  BS_Control12/1 -> MREPIsolationCockEnd2/1(InputControl)  "<MREPIsolationCockEnd2>"
  MREPIsolationCockEnd2/1(InputState) -> BC_Inputs/12  "MREPIsolationCockEnd2"
  BS_Control13/1 -> EPIC/1(InputControl)  "<EPIC>"
  EPIC/1(InputState) -> BC_Inputs/13  "EPIC"
  BS_Control14/1 -> ASCOEnd1/1(InputControl)  "<ASCOEnd1>"
  ASCOEnd1/1(InputState) -> BC_Inputs/14  "ASCOEnd1"
  BS_Control15/1 -> ASCOEnd2/1(InputControl)  "<ASCOEnd2>"
  ASCOEnd2/1(InputState) -> BC_Inputs/15  "ASCOEnd2"
  BS_Control16/1 -> ASIsolationCock/1(InputControl)  "<ASIsolationCock>"
  ASIsolationCock/1(InputState) -> BC_Inputs/16  "ASIsolationCock"
  BS_Control17/1 -> SR/1(InputControl)  "<SR>"
  SR/1(InputState) -> BC_Inputs/17  "SR"
  BS_Control18/1 -> ParkingBrakeManualReleaseBogie1Handle1/1(InputControl)  "<ParkingBrakeManualReleaseBogie1Handle1>"
  ParkingBrakeManualReleaseBogie1Handle1/1(InputState) -> BC_Inputs/18  "ParkingBrakeManualReleaseBogie1Handle1"
  BS_Control19/1 -> ParkingBrakeManualReleaseBogie1Handle2/1(InputControl)  "<ParkingBrakeManualReleaseBogie1Handle2>"
  ParkingBrakeManualReleaseBogie1Handle2/1(InputState) -> BC_Inputs/19  "ParkingBrakeManualReleaseBogie1Handle2"
  BS_Control20/1 -> ParkingBrakeManualReleaseBogie2Handle1/1(InputControl)  "<ParkingBrakeManualReleaseBogie2Handle1>"
  ParkingBrakeManualReleaseBogie2Handle1/1(InputState) -> BC_Inputs/20  "ParkingBrakeManualReleaseBogie2Handle1"
  BS_Control21/1 -> ParkingBrakeManualReleaseBogie2Handle2/1(InputControl)  "<ParkingBrakeManualReleaseBogie2Handle2>"
  ParkingBrakeManualReleaseBogie2Handle2/1(InputState) -> BC_Inputs/21  "ParkingBrakeManualReleaseBogie2Handle2"

== system IOControls/ForEachVehicle/IOControls/CabControl/DriverDesk/Gauges ==
  ModelInputs : Inport
  Initialise : Inport  Port=2
  BC_Inputs : BusCreator  Inputs=1
  BC_MCBTrip : BusCreator  Inputs=1
  InitialiseTerminator : Terminator
  InputsGround : Ground
  MCBTripGround : Ground
  ModelInputsTerminator : Terminator
  TierControlsInputs : Outport  VectorParamsAs1DForOutWhenUnconnected=off
  TierControlsMCBTrip : Outport  Port=2  VectorParamsAs1DForOutWhenUnconnected=off
  wires:
  MCBTripGround/1 -> BC_MCBTrip/1
  InputsGround/1 -> BC_Inputs/1
  Initialise/1 -> InitialiseTerminator/1
  ModelInputs/1 -> ModelInputsTerminator/1
  BC_MCBTrip/1 -> TierControlsMCBTrip/1  "Gauges"
  BC_Inputs/1 -> TierControlsInputs/1  "Gauges"

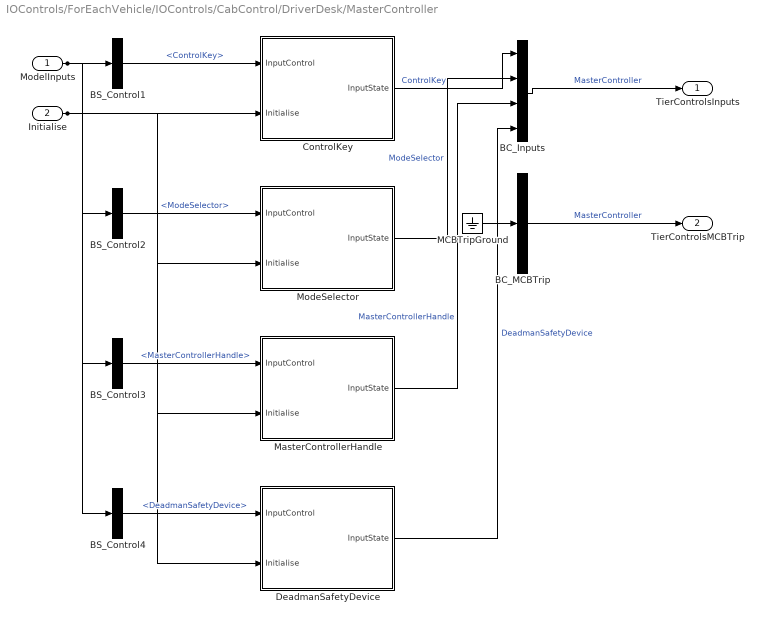
== system IOControls/ForEachVehicle/IOControls/CabControl/DriverDesk/MasterController ==
  ModelInputs : Inport
  Initialise : Inport  Port=2
  BC_Inputs : BusCreator  Inputs=4
  BC_MCBTrip : BusCreator  Inputs=1
  BS_Control1 : BusSelector  OutputSignals=ControlKey
  BS_Control2 : BusSelector  OutputSignals=ModeSelector
  BS_Control3 : BusSelector  OutputSignals=MasterControllerHandle
  BS_Control4 : BusSelector  OutputSignals=DeadmanSafetyDevice
  ControlKey : Subsystem  mask{InitState=0, ControlStates=[0,1], OnStateValue=1, OffStateValue=0}
      mask prompts: InitState "Initial State"; ControlStates "Software State Values"; OnStateValue "On State Value"; OffStateValue "Off State Value"
  DeadmanSafetyDevice : Subsystem  mask{InitState=0, ControlStates=[0,1], OnStateValue=1, OffStateValue=0}
      mask prompts: InitState "Initial State"; ControlStates "Software State Values"; OnStateValue "On State Value"; OffStateValue "Off State Value"
  MCBTripGround : Ground
  MasterControllerHandle : Subsystem  mask{InitState=-100, ControlStates=[-101,-100,-90,-80,-70,-60,-50,-40,-30,-20,-10,0,10,20,30,40,50,60,70,80,90,100], OnStateValue=100, OffStateValue=101}
      mask prompts: InitState "Initial State"; ControlStates "Software State Values"; OnStateValue "On State Value"; OffStateValue "Off State Value"
  ModeSelector : Subsystem  mask{InitState=0, ControlStates=[0,1,2,3,4,5], OnStateValue=5, OffStateValue=0}
      mask prompts: InitState "Initial State"; ControlStates "Software State Values"; OnStateValue "On State Value"; OffStateValue "Off State Value"
  TierControlsInputs : Outport  VectorParamsAs1DForOutWhenUnconnected=off
  TierControlsMCBTrip : Outport  Port=2  VectorParamsAs1DForOutWhenUnconnected=off
  wires:
  MCBTripGround/1 -> BC_MCBTrip/1
  BC_MCBTrip/1 -> TierControlsMCBTrip/1  "MasterController"
  BC_Inputs/1 -> TierControlsInputs/1  "MasterController"
  ModelInputs/1 -> BS_Control1/1, BS_Control2/1, BS_Control3/1, BS_Control4/1
  BS_Control1/1 -> ControlKey/1(InputControl)  "<ControlKey>"
  Initialise/1 -> ControlKey/2(Initialise), ModeSelector/2(Initialise), MasterControllerHandle/2(Initialise), DeadmanSafetyDevice/2(Initialise)
  ControlKey/1(InputState) -> BC_Inputs/1  "ControlKey"
  BS_Control2/1 -> ModeSelector/1(InputControl)  "<ModeSelector>"
  ModeSelector/1(InputState) -> BC_Inputs/2  "ModeSelector"
  BS_Control3/1 -> MasterControllerHandle/1(InputControl)  "<MasterControllerHandle>"
  MasterControllerHandle/1(InputState) -> BC_Inputs/3  "MasterControllerHandle"
  BS_Control4/1 -> DeadmanSafetyDevice/1(InputControl)  "<DeadmanSafetyDevice>"
  DeadmanSafetyDevice/1(InputState) -> BC_Inputs/4  "DeadmanSafetyDevice"
